simulink model "Fuzzy without derivative"  (R2022a)
settings: Solver=VariableStepAuto  StartTime=0.0  StopTime=20  RelTol=1e-3
libraries: fuzblock x1
settings Model: Creator=SEBASTIANDIAZPABON  LastModifiedBy=SEBASTIANDIAZPABON

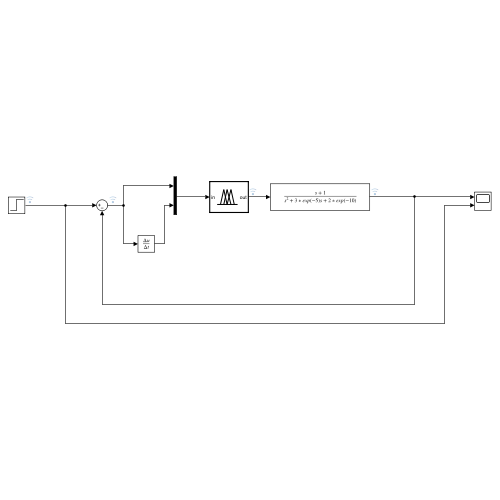
[thumbnail: Simulink's stored preview of the top-level diagram]
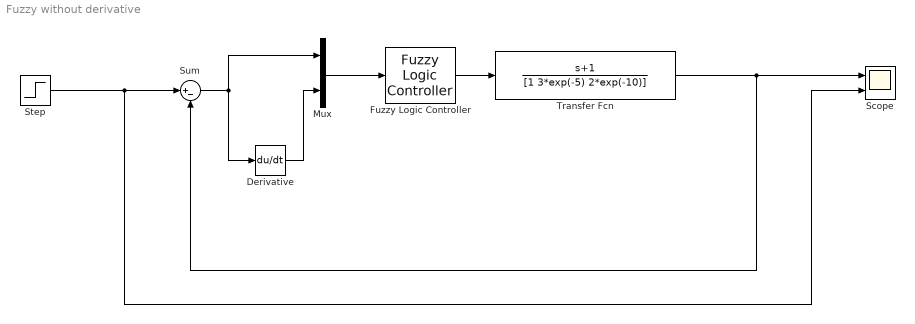
== system Fuzzy without derivative ==
  Derivative : Derivative
  Fuzzy Logic Controller : fuzblock/Fuzzy Logic  Controller  FIS='controller'  OutputSampleNumber=101  DataType=double  FuzzifiedInputs=off  RuleFiringStrengths=off  RuleOutputs=off  AggregatedOutputs=off  SimulateUsing=Interpreted execution  OutOfRangeInputValueMessage=warning  NoRuleFiredMessage=warning  EmptyOutputFuzzySetMessage=warning
  Mux : Mux  Inputs=2
  Scope : Scope  NumInputPorts=2
  Step : Step  After=0.1  SampleTime=0
  Sum : Sum  Inputs=|+-
  Transfer Fcn : TransferFcn  Numerator=[1 1]  Denominator=[1 3*exp(-5) 2*exp(-10)]
  wires:
  Transfer Fcn/1 -> Sum/2, Scope/1
  Step/1 -> Scope/2, Sum/1
  Sum/1 -> Mux/1, Derivative/1
  Fuzzy Logic Controller/1 -> Transfer Fcn/1
  Mux/1 -> Fuzzy Logic Controller/1
  Derivative/1 -> Mux/2
